simulink library "wndlib2"  (Simulink 2.09)
libraries: wndlib2 x6

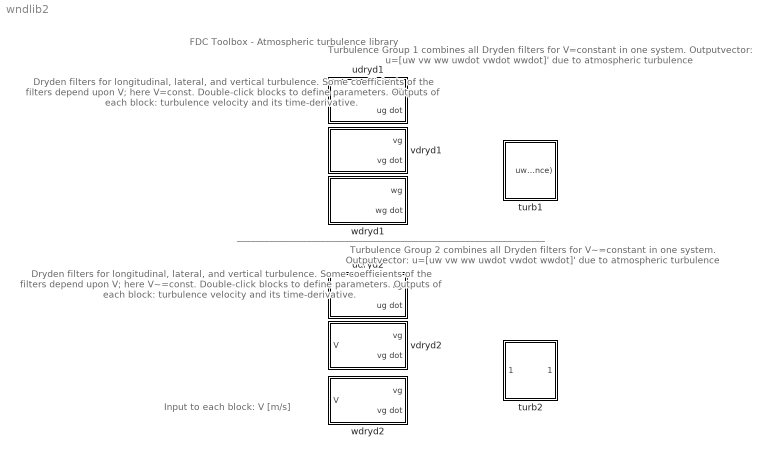
== system wndlib2 ==
  note: FDC Toolbox - Atmospheric turbulence library
  note: Turbulence Group 2 combines
      | all Dryden filters for V~=constant in
      | one system. Outputvector:
      | u=[uw vw ww uwdot vwdot wwdot]'
      | due to atmospheric turbulence
  note: Input to each block: V [m/s]
  note: Dryden filters for longitudinal,
      | lateral, and vertical turbulence.
      | Some coefficients of the filters
      | depend upon V; here V~=const.
      |
      | Double-click blocks to define
      | parameters. Outputs of each
      | block: turbulence velocity
      | and its time-derivative.
  note: __________________________________________________________________
  note: Dryden filters for longitudinal,
      | lateral, and vertical turbulence.
      | Some coefficients of the filters
      | depend upon V; here V=const.
      |
      | Double-click blocks to define
      | parameters. Outputs of each
      | block: turbulence velocity
      | and its time-derivative.
  note: Turbulence Group 1 combines
      | all Dryden filters for V=constant in
      | one system. Outputvector:
      | u=[uw vw ww uwdot vwdot wwdot]'
      | due to atmospheric turbulence
  turb1 : Subsystem
  turb2 : Subsystem
  "udryd1 " : Subsystem  mask(udryd1){@1=150, @2=1, @3=45}
      mask prompts: @1 "Scale length Lug [m]:"; @2 "Standard deviation sigma_ug [m/s]:"; @3 "TAS [m/s]:"
      mask help:
      | Longitudinal Dryden filter
      | V=const
      mask init:
      | K = @2*sqrt(2*@1/@3); tau = @1/@3;
      mask Help: eval('fdchelp udryd1')
      mask Display: disp('Longitudinal\nDryden filter\nV=const')
  "udryd2 " : Subsystem  mask(udryd2){Lug=150, sigma_ug=1}
      mask prompts: Lug "Scale length Lug [m]:"; sigma_ug "Standard deviation sigma_ug [m/s]:"
      mask help:
      | Longitudinal Dryden filter with
      | coefficients which vary with V
      mask Help: eval('fdchelp udryd2')
      mask Display: disp('Longitudinal\nDryden filter\nV~=const')
  "vdryd1 " : Subsystem  mask(vdryd1){@1=150, @2=1, @3=45}
      mask prompts: @1 "Scale length Lvg [m]:"; @2 "Standard deviation sigma_vg [m/s]:"; @3 "True airspeed [m/s]:"
      mask help:
      | Lateral Dryden filter
      | V=const
      mask init:
      | VL=@3/@1; a0=VL^2; a1=2*VL; b0=@2*sqrt(1/VL)*VL^2; b1=@2*sqrt(3/VL)*VL;
      mask Help: eval('fdchelp vdryd1')
      mask Display: disp('Lateral\nDryden filter\nV=const')
  "vdryd2 " : Subsystem  mask(vdryd2){Lvg=150, sigma_vg=1}
      mask prompts: Lvg "Scale length Lvg [m]:"; sigma_vg "Standard deviation sigma_vg [m/s]:"
      mask help:
      | Lateral Dryden filter with
      | coefficients which vary with V
      mask Help: eval('fdchelp vdryd2')
      mask Display: disp('Lateral\nDryden filter\nV~=const')
  "wdryd1 " : Subsystem  mask(wdryd1){@1=150, @2=1, @3=45}
      mask prompts: @1 "Scale length Lwg [m]:"; @2 "Standard deviation sigma_wg [m/s]:"; @3 "True airspeed [m/s]:"
      mask help:
      | Vertical Dryden filter
      | V=const
      mask init:
      | VL=@3/@1; a0=VL^2; a1=2*VL; b0=@2*sqrt(1/VL)*VL^2; b1=@2*sqrt(3/VL)*VL;
      mask Help: eval('fdchelp wdryd1')
      mask Display: disp('Vertical\nDryden filter\nV=const')
  "wdryd2 " : Subsystem  mask(wdryd2){Lwg=150, sigma_wg=1}
      mask prompts: Lwg "Scale length Lwg [m]:"; sigma_wg "Standard deviation sigma_wg [m/s]:"
      mask help:
      | Vertical Dryden filter with
      | coefficients which vary with V
      mask Help: eval('fdchelp wdryd2')
      mask Display: disp('Vertical\nDryden filter\nV~=const')

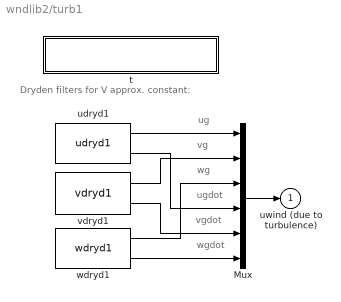
== system wndlib2/turb1 ==
  note: wgdot
  note: vgdot
  note: ugdot
  note: wg
  note: vg
  note: ug
  note: Dryden filters for V
      | approx. constant:
  Mux : Mux  Inputs=6
  t : Subsystem
      settings: OpenFcn=fdchelp turb1
      mask Display: disp('Atmospheric Turbulence Group 1\nMarc Rauw')
  "udryd1 " : wndlib2/udryd1   MaskParam1=150  MaskParam2=1  MaskParam3=45
  "vdryd1 " : wndlib2/vdryd1   MaskParam1=150  MaskParam2=1  MaskParam3=45
  "wdryd1 " : wndlib2/wdryd1   MaskParam1=150  MaskParam2=1  MaskParam3=45
  uwind (due to turbulence) : Outport  Port=1  InitialOutput=0
  wires:
  "vdryd1 "/1 -> Mux/2
  Mux/1 -> uwind (due to turbulence)/1
  "vdryd1 "/2 -> Mux/5
  "wdryd1 "/1 -> Mux/3
  "wdryd1 "/2 -> Mux/6
  "udryd1 "/2 -> Mux/4
  "udryd1 "/1 -> Mux/1

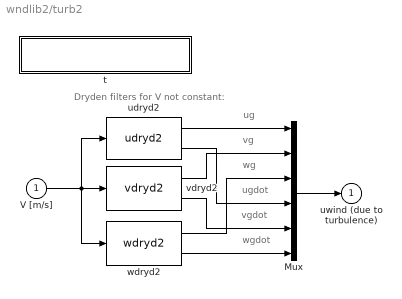
== system wndlib2/turb2 ==
  note: wgdot
  note: vgdot
  note: ugdot
  note: wg
  note: vg
  note: ug
  note: Dryden filters for
      | V not constant:
  V [m/s] : Inport  Port=1  PortWidth=-1  SampleTime=-1
  Mux : Mux  Inputs=6
  t : Subsystem
      settings: OpenFcn=fdchelp turb2
      mask Display: disp('Atmospheric Turbulence Group 2\nMarc Rauw')
  "udryd2 " : wndlib2/udryd2   Lug=150  sigma_ug=1
  "vdryd2 " : wndlib2/vdryd2   Lvg=150  sigma_vg=1
  "wdryd2 " : wndlib2/wdryd2   Lwg=150  sigma_wg=1
  uwind (due to turbulence) : Outport  Port=1  InitialOutput=0
  wires:
  V [m/s]/1 -> "wdryd2 "/1, "udryd2 "/1, "vdryd2 "/1
  Mux/1 -> uwind (due to turbulence)/1
  "vdryd2 "/2 -> Mux/5
  "vdryd2 "/1 -> Mux/2
  "wdryd2 "/1 -> Mux/3
  "wdryd2 "/2 -> Mux/6
  "udryd2 "/2 -> Mux/4
  "udryd2 "/1 -> Mux/1

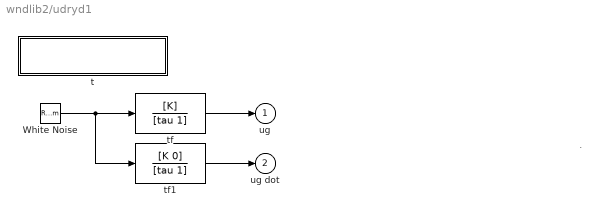
== system wndlib2/udryd1  ==
  note: .
  White Noise : RandomNumber  Mean=0  Variance=1  Seed=0  SampleTime=-1
  t : Subsystem
      settings: OpenFcn=fdchelp udryd1
      mask Display: disp('Longitudinal Dryden filter\nMarc Rauw, October 1997')
  tf : TransferFcn  Numerator=[K]  Denominator=[tau 1]
  tf1 : TransferFcn  Numerator=[K 0]  Denominator=[tau 1]
  ug : Outport  Port=1  InitialOutput=0
  ug dot : Outport  Port=2  InitialOutput=0
  wires:
  tf1/1 -> ug dot/1
  White Noise/1 -> tf1/1, tf/1
  tf/1 -> ug/1

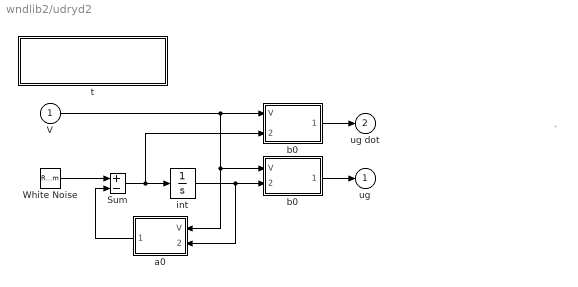
== system wndlib2/udryd2  ==
  note: `
  V : Inport  Port=1  PortWidth=-1  SampleTime=-1
  Sum : Sum  Inputs=+-
  White Noise : RandomNumber  Mean=0  Variance=1  Seed=0  SampleTime=-1
  a0 : Subsystem  Orientation=left
      mask Display: plot(0,0,100,100,[100,0,100],[0,50,100]);disp('       K(u1)')
  b0 : Subsystem
      mask Display: plot(0,0,100,100,[0,100,0],[0,50,100]);disp('K(u1)      ')
  "b0 " : Subsystem
      mask Display: plot(0,0,100,100,[0,100,0],[0,50,100]);disp('K(u1)      ')
  int : Integrator  ExternalReset=none  InitialConditionSource=internal  InitialCondition=0  LimitOutput=off  UpperSaturationLimit=inf  LowerSaturationLimit=-inf  ShowSaturationPort=off  ShowStatePort=off  AbsoluteTolerance=auto
  t : Subsystem
      settings: OpenFcn=fdchelp udryd2
      mask Display: disp('Longitudinal Dryden filter\n(coefficients vary with V)\nMarc Rauw, October 1997')
  ug : Outport  Port=1  InitialOutput=0
  ug dot : Outport  Port=2  InitialOutput=0
  wires:
  b0/1(y = K*u) -> ug/1
  int/1 -> a0/2(input u), b0/2(input u)
  a0/1(y = K*u) -> Sum/2
  White Noise/1 -> Sum/1
  Sum/1 -> "b0 "/2(input u), int/1
  V/1 -> b0/1(V), a0/1(V), "b0 "/1(V)
  "b0 "/1(y = K*u) -> ug dot/1

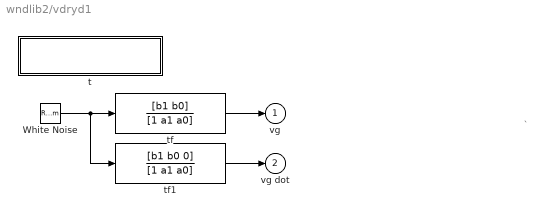
== system wndlib2/vdryd1  ==
  note: `
  White Noise : RandomNumber  Mean=0  Variance=1  Seed=10  SampleTime=-1
  t : Subsystem
      settings: OpenFcn=fdchelp vdryd1
      mask Display: disp('Lateral Dryden filter\nMarc Rauw, October 1997')
  tf : TransferFcn  Numerator=[b1 b0]  Denominator=[1 a1 a0]
  tf1 : TransferFcn  Numerator=[b1 b0 0]  Denominator=[1 a1 a0]
  vg : Outport  Port=1  InitialOutput=0
  vg dot : Outport  Port=2  InitialOutput=0
  wires:
  White Noise/1 -> tf1/1, tf/1
  tf1/1 -> vg dot/1
  tf/1 -> vg/1

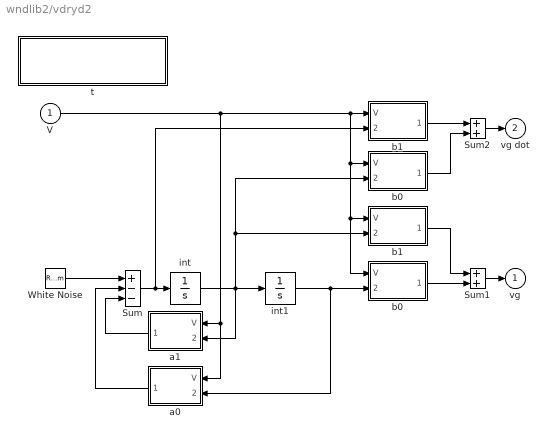
== system wndlib2/vdryd2  ==
  V : Inport  Port=1  PortWidth=-1  SampleTime=-1
  Sum : Sum  Inputs=+--
  Sum1 : Sum  Inputs=++
  Sum2 : Sum  Inputs=++
  White Noise : RandomNumber  Mean=0  Variance=1  Seed=10  SampleTime=-1
  a0 : Subsystem  Orientation=left
      mask Display: plot(0,0,100,100,[100,0,100],[0,50,100]);disp('       K(u1)')
  a1 : Subsystem  Orientation=left
      mask Display: plot(0,0,100,100,[100,0,100],[0,50,100]);disp('       K(u1)')
  b0 : Subsystem
      mask Display: plot(0,0,100,100,[0,100,0],[0,50,100]);disp('K(u1)      ')
  "b0 " : Subsystem
      mask Display: plot(0,0,100,100,[0,100,0],[0,50,100]);disp('K(u1)      ')
  b1 : Subsystem
      mask Display: plot(0,0,100,100,[0,100,0],[0,50,100]);disp('K(u1)      ')
  "b1 " : Subsystem
      mask Display: plot(0,0,100,100,[0,100,0],[0,50,100]);disp('K(u1)      ')
  int : Integrator  ExternalReset=none  InitialConditionSource=internal  InitialCondition=0  LimitOutput=off  UpperSaturationLimit=inf  LowerSaturationLimit=-inf  ShowSaturationPort=off  ShowStatePort=off  AbsoluteTolerance=auto
  int1 : Integrator  ExternalReset=none  InitialConditionSource=internal  InitialCondition=0  LimitOutput=off  UpperSaturationLimit=inf  LowerSaturationLimit=-inf  ShowSaturationPort=off  ShowStatePort=off  AbsoluteTolerance=auto
  t : Subsystem
      settings: OpenFcn=fdchelp vdryd2
      mask Display: disp('Lateral Dryden filter\n(coefficients vary with V)\nMarc Rauw, October 1997')
  vg : Outport  Port=1  InitialOutput=0
  vg dot : Outport  Port=2  InitialOutput=0
  wires:
  V/1 -> a1/1(V), a0/1(V), b1/1(V), b0/1(V), "b0 "/1(V), "b1 "/1(V)
  White Noise/1 -> Sum/1
  int1/1 -> a0/2(input u), b0/2(input u)
  a0/1(y = K*u) -> Sum/2
  a1/1(y = K*u) -> Sum/3
  b1/1(y = K*u) -> Sum1/1
  b0/1(y = K*u) -> Sum1/2
  Sum1/1 -> vg/1
  Sum2/1 -> vg dot/1
  "b1 "/1(y = K*u) -> Sum2/1
  "b0 "/1(y = K*u) -> Sum2/2
  Sum/1 -> "b1 "/2(input u), int/1
  int/1 -> a1/2(input u), "b0 "/2(input u), b1/2(input u), int1/1

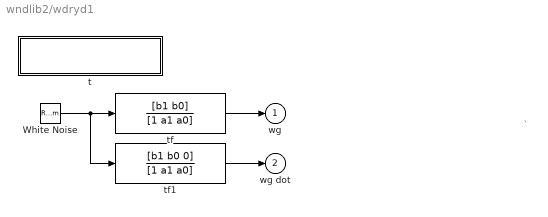
== system wndlib2/wdryd1  ==
  note: `
  White Noise : RandomNumber  Mean=0  Variance=1  Seed=20  SampleTime=-1
  t : Subsystem
      settings: OpenFcn=fdchelp wdryd1
      mask Display: disp('Vertical Dryden filter\nMarc Rauw, October 1997')
  tf : TransferFcn  Numerator=[b1 b0]  Denominator=[1 a1 a0]
  tf1 : TransferFcn  Numerator=[b1 b0 0]  Denominator=[1 a1 a0]
  wg : Outport  Port=1  InitialOutput=0
  wg dot : Outport  Port=2  InitialOutput=0
  wires:
  tf/1 -> wg/1
  tf1/1 -> wg dot/1
  White Noise/1 -> tf1/1, tf/1

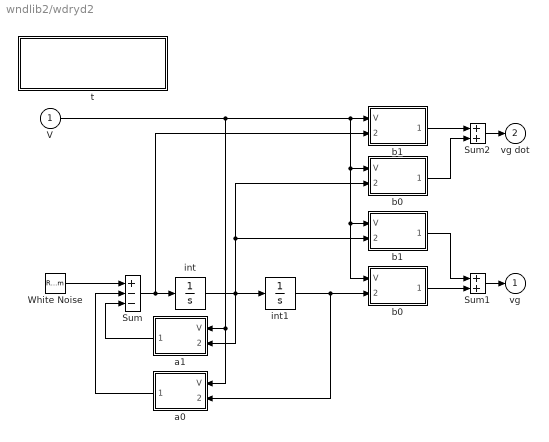
== system wndlib2/wdryd2  ==
  V : Inport  Port=1  PortWidth=-1  SampleTime=-1
  Sum : Sum  Inputs=+--
  Sum1 : Sum  Inputs=++
  Sum2 : Sum  Inputs=++
  White Noise : RandomNumber  Mean=0  Variance=1  Seed=20  SampleTime=-1
  a0 : Subsystem  Orientation=left
      mask Display: plot(0,0,100,100,[100,0,100],[0,50,100]);disp('       K(u1)')
  a1 : Subsystem  Orientation=left
      mask Display: plot(0,0,100,100,[100,0,100],[0,50,100]);disp('       K(u1)')
  b0 : Subsystem
      mask Display: plot(0,0,100,100,[0,100,0],[0,50,100]);disp('K(u1)      ')
  "b0 " : Subsystem
      mask Display: plot(0,0,100,100,[0,100,0],[0,50,100]);disp('K(u1)      ')
  b1 : Subsystem
      mask Display: plot(0,0,100,100,[0,100,0],[0,50,100]);disp('K(u1)      ')
  "b1 " : Subsystem
      mask Display: plot(0,0,100,100,[0,100,0],[0,50,100]);disp('K(u1)      ')
  int : Integrator  ExternalReset=none  InitialConditionSource=internal  InitialCondition=0  LimitOutput=off  UpperSaturationLimit=inf  LowerSaturationLimit=-inf  ShowSaturationPort=off  ShowStatePort=off  AbsoluteTolerance=auto
  int1 : Integrator  ExternalReset=none  InitialConditionSource=internal  InitialCondition=0  LimitOutput=off  UpperSaturationLimit=inf  LowerSaturationLimit=-inf  ShowSaturationPort=off  ShowStatePort=off  AbsoluteTolerance=auto
  t : Subsystem
      settings: OpenFcn=fdchelp wdryd2
      mask Display: disp('Vertical Dryden filter\n(coefficients vary with V)\nMarc Rauw, October 1997')
  vg : Outport  Port=1  InitialOutput=0
  vg dot : Outport  Port=2  InitialOutput=0
  wires:
  Sum/1 -> "b1 "/2(input u), int/1
  "b0 "/1(y = K*u) -> Sum2/2
  "b1 "/1(y = K*u) -> Sum2/1
  Sum2/1 -> vg dot/1
  Sum1/1 -> vg/1
  b0/1(y = K*u) -> Sum1/2
  b1/1(y = K*u) -> Sum1/1
  a1/1(y = K*u) -> Sum/3
  a0/1(y = K*u) -> Sum/2
  int/1 -> "b0 "/2(input u), b1/2(input u), a1/2(input u), int1/1
  int1/1 -> a0/2(input u), b0/2(input u)
  V/1 -> a0/1(V), a1/1(V), "b0 "/1(V), b1/1(V), b0/1(V), "b1 "/1(V)
  White Noise/1 -> Sum/1

== system wndlib2/turb1/t ==

== system wndlib2/turb2/t ==

== system wndlib2/udryd1 /t ==

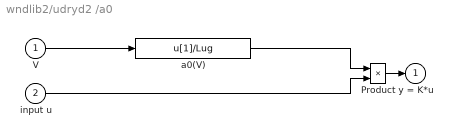
== system wndlib2/udryd2 /a0 ==
  V : Inport  Port=1  PortWidth=-1  SampleTime=-1
  input u : Inport  Port=2  PortWidth=-1  SampleTime=-1
  Product : Product  Inputs=2
  a0(V) : Fcn  Expr=u[1]/Lug
  y = K*u : Outport  Port=1  InitialOutput=0
  wires:
  V/1 -> a0(V)/1
  Product/1 -> y = K*u/1
  input u/1 -> Product/2
  a0(V)/1 -> Product/1

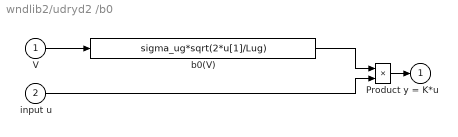
== system wndlib2/udryd2 /b0 ==
  V : Inport  Port=1  PortWidth=-1  SampleTime=-1
  input u : Inport  Port=2  PortWidth=-1  SampleTime=-1
  Product : Product  Inputs=2
  b0(V) : Fcn  Expr=sigma_ug*sqrt(2*u[1]/Lug)
  y = K*u : Outport  Port=1  InitialOutput=0
  wires:
  V/1 -> b0(V)/1
  Product/1 -> y = K*u/1
  input u/1 -> Product/2
  b0(V)/1 -> Product/1

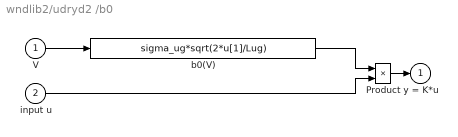
== system wndlib2/udryd2 /b0  ==
  V : Inport  Port=1  PortWidth=-1  SampleTime=-1
  input u : Inport  Port=2  PortWidth=-1  SampleTime=-1
  Product : Product  Inputs=2
  b0(V) : Fcn  Expr=sigma_ug*sqrt(2*u[1]/Lug)
  y = K*u : Outport  Port=1  InitialOutput=0
  wires:
  b0(V)/1 -> Product/1
  input u/1 -> Product/2
  Product/1 -> y = K*u/1
  V/1 -> b0(V)/1

== system wndlib2/udryd2 /t ==

== system wndlib2/vdryd1 /t ==

== system wndlib2/vdryd2 /a0 ==
  V : Inport  Port=1  PortWidth=-1  SampleTime=-1
  input u : Inport  Port=2  PortWidth=-1  SampleTime=-1
  Product : Product  Inputs=2
  a0(V) : Fcn  Expr=(u[1]/Lvg)^2
  y = K*u : Outport  Port=1  InitialOutput=0
  wires:
  a0(V)/1 -> Product/1
  input u/1 -> Product/2
  Product/1 -> y = K*u/1
  V/1 -> a0(V)/1

== system wndlib2/vdryd2 /a1 ==
  V : Inport  Port=1  PortWidth=-1  SampleTime=-1
  input u : Inport  Port=2  PortWidth=-1  SampleTime=-1
  Product : Product  Inputs=2
  a1(V) : Fcn  Expr=2*(u[1]/Lvg)
  y = K*u : Outport  Port=1  InitialOutput=0
  wires:
  V/1 -> a1(V)/1
  Product/1 -> y = K*u/1
  input u/1 -> Product/2
  a1(V)/1 -> Product/1

== system wndlib2/vdryd2 /b0 ==
  V : Inport  Port=1  PortWidth=-1  SampleTime=-1
  input u : Inport  Port=2  PortWidth=-1  SampleTime=-1
  Product : Product  Inputs=2
  b0(V) : Fcn  Expr=sigma_vg*sqrt(Lvg/u[1])*(u[1]/Lvg)^2
  y = K*u : Outport  Port=1  InitialOutput=0
  wires:
  input u/1 -> Product/2
  b0(V)/1 -> Product/1
  Product/1 -> y = K*u/1
  V/1 -> b0(V)/1

== system wndlib2/vdryd2 /b0  ==
  V : Inport  Port=1  PortWidth=-1  SampleTime=-1
  input u : Inport  Port=2  PortWidth=-1  SampleTime=-1
  Product : Product  Inputs=2
  b0(V) : Fcn  Expr=sigma_vg*sqrt(Lvg/u[1])*(u[1]/Lvg)^2
  y = K*u : Outport  Port=1  InitialOutput=0
  wires:
  input u/1 -> Product/2
  b0(V)/1 -> Product/1
  Product/1 -> y = K*u/1
  V/1 -> b0(V)/1

== system wndlib2/vdryd2 /b1 ==
  V : Inport  Port=1  PortWidth=-1  SampleTime=-1
  input u : Inport  Port=2  PortWidth=-1  SampleTime=-1
  Product : Product  Inputs=2
  b0(V) : Fcn  Expr=sigma_vg*sqrt(3*Lvg/u[1])*(u[1]/Lvg)
  y = K*u : Outport  Port=1  InitialOutput=0
  wires:
  b0(V)/1 -> Product/1
  V/1 -> b0(V)/1
  Product/1 -> y = K*u/1
  input u/1 -> Product/2

== system wndlib2/vdryd2 /b1  ==
  V : Inport  Port=1  PortWidth=-1  SampleTime=-1
  input u : Inport  Port=2  PortWidth=-1  SampleTime=-1
  Product : Product  Inputs=2
  b0(V) : Fcn  Expr=sigma_vg*sqrt(3*Lvg/u[1])*(u[1]/Lvg)
  y = K*u : Outport  Port=1  InitialOutput=0
  wires:
  b0(V)/1 -> Product/1
  input u/1 -> Product/2
  Product/1 -> y = K*u/1
  V/1 -> b0(V)/1

== system wndlib2/vdryd2 /t ==

== system wndlib2/wdryd1 /t ==

== system wndlib2/wdryd2 /a0 ==
  V : Inport  Port=1  PortWidth=-1  SampleTime=-1
  input u : Inport  Port=2  PortWidth=-1  SampleTime=-1
  Product : Product  Inputs=2
  a0(V) : Fcn  Expr=(u[1]/Lwg)^2
  y = K*u : Outport  Port=1  InitialOutput=0
  wires:
  V/1 -> a0(V)/1
  Product/1 -> y = K*u/1
  a0(V)/1 -> Product/1
  input u/1 -> Product/2

== system wndlib2/wdryd2 /a1 ==
  V : Inport  Port=1  PortWidth=-1  SampleTime=-1
  input u : Inport  Port=2  PortWidth=-1  SampleTime=-1
  Product : Product  Inputs=2
  a1(V) : Fcn  Expr=2*(u[1]/Lwg)
  y = K*u : Outport  Port=1  InitialOutput=0
  wires:
  input u/1 -> Product/2
  a1(V)/1 -> Product/1
  Product/1 -> y = K*u/1
  V/1 -> a1(V)/1

== system wndlib2/wdryd2 /b0 ==
  V : Inport  Port=1  PortWidth=-1  SampleTime=-1
  input u : Inport  Port=2  PortWidth=-1  SampleTime=-1
  Product : Product  Inputs=2
  b0(V) : Fcn  Expr=sigma_wg*sqrt(Lwg/u[1])*(u[1]/Lwg)^2
  y = K*u : Outport  Port=1  InitialOutput=0
  wires:
  V/1 -> b0(V)/1
  Product/1 -> y = K*u/1
  input u/1 -> Product/2
  b0(V)/1 -> Product/1

== system wndlib2/wdryd2 /b0  ==
  V : Inport  Port=1  PortWidth=-1  SampleTime=-1
  input u : Inport  Port=2  PortWidth=-1  SampleTime=-1
  Product : Product  Inputs=2
  b0(V) : Fcn  Expr=sigma_wg*sqrt(Lwg/u[1])*(u[1]/Lwg)^2
  y = K*u : Outport  Port=1  InitialOutput=0
  wires:
  V/1 -> b0(V)/1
  Product/1 -> y = K*u/1
  input u/1 -> Product/2
  b0(V)/1 -> Product/1

== system wndlib2/wdryd2 /b1 ==
  V : Inport  Port=1  PortWidth=-1  SampleTime=-1
  input u : Inport  Port=2  PortWidth=-1  SampleTime=-1
  Product : Product  Inputs=2
  b0(V) : Fcn  Expr=sigma_wg*sqrt(3*Lwg/u[1])*(u[1]/Lwg)
  y = K*u : Outport  Port=1  InitialOutput=0
  wires:
  b0(V)/1 -> Product/1
  input u/1 -> Product/2
  Product/1 -> y = K*u/1
  V/1 -> b0(V)/1

== system wndlib2/wdryd2 /b1  ==
  V : Inport  Port=1  PortWidth=-1  SampleTime=-1
  input u : Inport  Port=2  PortWidth=-1  SampleTime=-1
  Product : Product  Inputs=2
  b0(V) : Fcn  Expr=sigma_wg*sqrt(3*Lwg/u[1])*(u[1]/Lwg)
  y = K*u : Outport  Port=1  InitialOutput=0
  wires:
  V/1 -> b0(V)/1
  Product/1 -> y = K*u/1
  input u/1 -> Product/2
  b0(V)/1 -> Product/1

== system wndlib2/wdryd2 /t ==
